simulink model "Messwerte_Sync"  (R2021b)
settings: Solver=FixedStepAuto  StartTime=0.0  StopTime=max(ASMod_dmEGFld_3(:,1))  FixedStep=stepsize  RelTol=1e-3
settings Model: Creator=q552088  LastModifiedBy=q552088

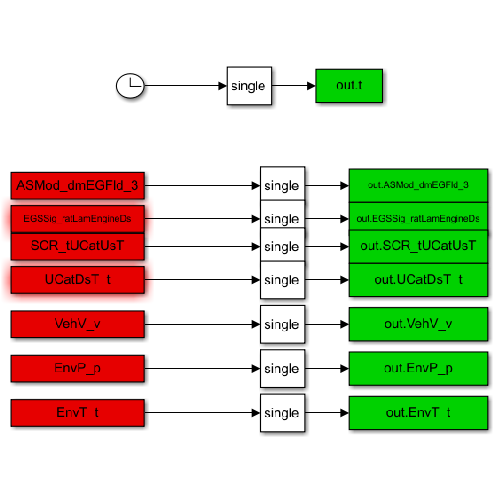
[thumbnail: Simulink's stored preview of the top-level diagram]
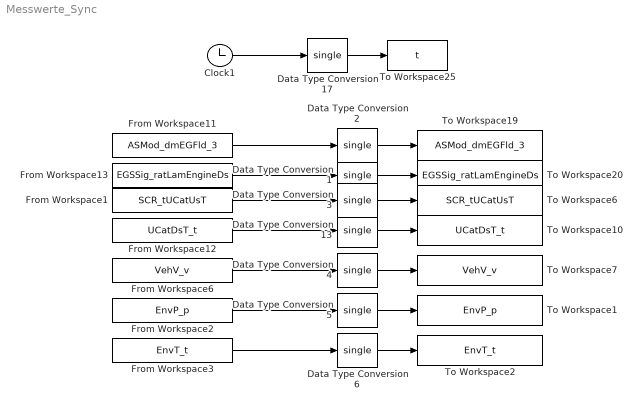
== system Messwerte_Sync ==
  Clock1 : Clock
  Data Type Conversion{1..6,13,17} (8 alike) : DataTypeConversion  OutDataTypeStr=single
  From Workspace1 : FromWorkspace  VariableName=SCR_tUCatUsT  Interpolate=off  OutputAfterFinalValue=Holding final value
  From Workspace11 : FromWorkspace  VariableName=ASMod_dmEGFld_3  Interpolate=off  OutputAfterFinalValue=Holding final value
  From Workspace12 : FromWorkspace  VariableName=UCatDsT_t  Interpolate=off  OutputAfterFinalValue=Holding final value
  From Workspace13 : FromWorkspace  VariableName=EGSSig_ratLamEngineDs  Interpolate=off  OutputAfterFinalValue=Holding final value
  From Workspace2 : FromWorkspace  VariableName=EnvP_p  Interpolate=off  OutputAfterFinalValue=Holding final value
  From Workspace3 : FromWorkspace  VariableName=EnvT_t  Interpolate=off  OutputAfterFinalValue=Holding final value
  From Workspace6 : FromWorkspace  VariableName=VehV_v  Interpolate=off  OutputAfterFinalValue=Holding final value
  To Workspace1 : ToWorkspace  VariableName=EnvP_p  SampleTime=-1
  To Workspace10 : ToWorkspace  VariableName=UCatDsT_t  SampleTime=-1
  To Workspace19 : ToWorkspace  VariableName=ASMod_dmEGFld_3  SampleTime=-1
  To Workspace2 : ToWorkspace  VariableName=EnvT_t  SampleTime=-1
  To Workspace20 : ToWorkspace  VariableName=EGSSig_ratLamEngineDs  SampleTime=-1
  To Workspace25 : ToWorkspace  VariableName=t  SampleTime=-1
  To Workspace6 : ToWorkspace  VariableName=SCR_tUCatUsT  SampleTime=-1
  To Workspace7 : ToWorkspace  VariableName=VehV_v  SampleTime=-1
  wires:
  Data Type Conversion3/1 -> To Workspace6/1
  From Workspace1/1 -> Data Type Conversion3/1
  From Workspace13/1 -> Data Type Conversion1/1
  Data Type Conversion1/1 -> To Workspace20/1
  Data Type Conversion17/1 -> To Workspace25/1
  Data Type Conversion2/1 -> To Workspace19/1
  Data Type Conversion4/1 -> To Workspace7/1
  From Workspace6/1 -> Data Type Conversion4/1
  Clock1/1 -> Data Type Conversion17/1
  From Workspace11/1 -> Data Type Conversion2/1
  From Workspace12/1 -> Data Type Conversion13/1
  Data Type Conversion13/1 -> To Workspace10/1
  From Workspace2/1 -> Data Type Conversion5/1
  Data Type Conversion5/1 -> To Workspace1/1
  From Workspace3/1 -> Data Type Conversion6/1
  Data Type Conversion6/1 -> To Workspace2/1
